simulink model "Es2_sim"  (R2018b)
settings: Solver=VariableStepAuto  StartTime=0.0  StopTime=5  RelTol=1e-3
libraries: simulink x1
settings Model: Creator=claudio  LastModifiedBy=utente
settings SFSimCC: SimUseLocalCustomCode=off
settings RTWCC: RTWUseLocalCustomCode=off

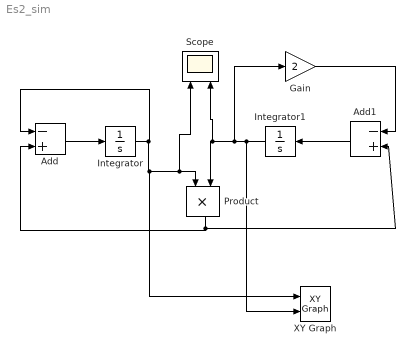
== system Es2_sim ==
  Add : Sum  Inputs=-+
  Add1 : Sum  Inputs=-+
  Gain : Gain  Gain=2
  Integrator : Integrator  InitialCondition=-30
  Integrator1 : Integrator  InitialCondition=-30
  Product : Product
  Scope : Scope  NumInputPorts=2
  XY Graph : simulink/Sinks/XY Graph  xmin=-50  xmax=50  ymin=-50  ymax=50  st=-1
  wires:
  Add/1 -> Integrator/1
  Integrator/1 -> XY Graph/1, Scope/1, Product/1, Add/1
  Integrator1/1 -> XY Graph/2, Gain/1, Scope/2, Product/2
  Product/1 -> Add1/2, Add/2
  Add1/1 -> Integrator1/1
  Gain/1 -> Add1/1
